simulink model "Transition"  (R2019a)
settings: Solver=VariableStepAuto  StartTime=0.0  StopTime=40  RelTol=1e-3
values from neighbouring files (symbols this model uses):
  agent = rlDDPGAgent(actor,critic,agentOptions)    [Agent.m]    (also in Bigger_Agent.m = agent.saved_agent; Multirotor_Agent.m = rlDDPGAgent(actor,critic,agentOpts); Transition_Agent.m = rlDDPGAgent(actor,critic,agentOpts))
  Ts = 0.4    [Agent.m]    (also in Bigger_Agent.m = 0.3; Multirotor_Agent.m = 0.3; Transition_Agent.m = 0.3)
libraries: simulink x14, simulink_extras x5, sharedutil x3, aerolibasang x2, shared6dof x1, aerolibadyn x1
(part 2 of 2)

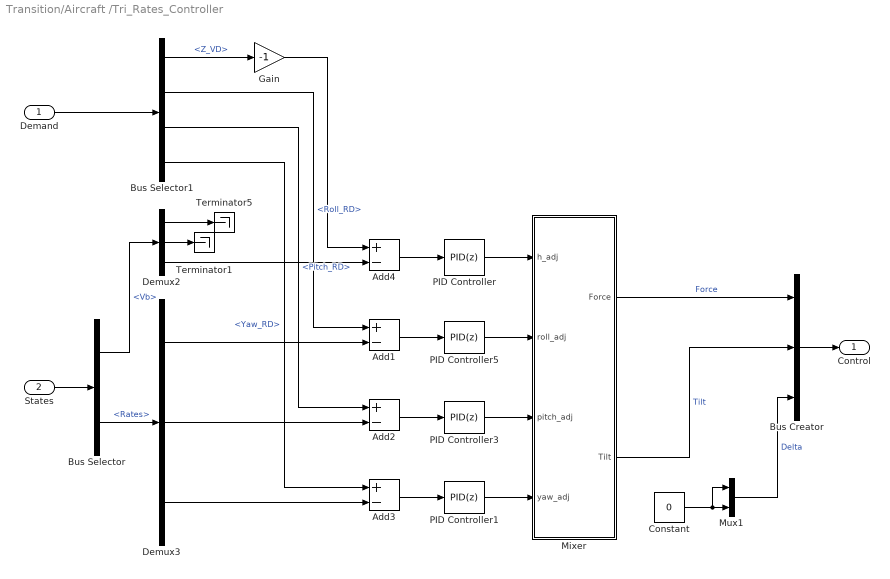
== system Transition/Aircraft /Tri_Rates_Controller ==
  Demand : Inport
  "States " : Inport  Port=2
  Add{1..4} (4 alike) : Sum  Inputs=+-
  Bus Creator : BusCreator  Inputs=3
  Bus Selector : BusSelector  OutputSignals=Vb,Rates
  Bus Selector1 : BusSelector  OutputSignals=Z_VD,Roll_RD,Pitch_RD,Yaw_RD
  Constant : Constant  Value=0
  Demux2 : Demux  Outputs=3
  Demux3 : Demux  Outputs=3
  Gain : Gain  Gain=-1
  Mixer : Subsystem
  Mux1 : Mux  Inputs=2
  PID Controller : simulink/Continuous/PID Controller  Controller=PID  Form=Parallel  TimeDomain=Discrete-time  SampleTime=0.001  IntegratorMethod=Forward Euler  FilterMethod=Forward Euler  ControllerParametersSource=internal  P=30  I=0.01  D=1  UseFilter=on  N=21.8158810168648  TunerSelectOption=Transfer Function Based (PID Tuner App)  InitialConditionSource=internal  InitialConditionForIntegrator=0  InitialConditionForFilter=0  DifferentiatorICPrevScaledInput=0  ExternalReset=none  TrackingMode=off  Kt=1  LimitOutput=off  UpperSaturationLimit=inf  LowerSaturationLimit=-inf  LinearizeAsGain=on  AntiWindupMode=none  Kb=1  POutMin=[]  POutMax=[]  IOutMin=[]  IOutMax=[]  DOutMin=[]  DOutMax=[]  NOutMin=[]  NOutMax=[]  SumOutMin=[]  SumOutMax=[]  SaturationOutMin=[]  SaturationOutMax=[]  PParamMin=[]  PParamMax=[]  IParamMin=[]  IParamMax=[]  DParamMin=[]  DParamMax=[]  NParamMin=[]  NParamMax=[]  KbParamMin=[]  KbParamMax=[]  KtParamMin=[]  KtParamMax=[]  KbOutMin=[]  KbOutMax=[]  KtOutMin=[]  KtOutMax=[]  IntegratorOutMin=[]  IntegratorOutMax=[]  FilterOutMin=[]  FilterOutMax=[]  SumI1OutMin=[]  SumI1OutMax=[]  SumI2OutMin=[]  SumI2OutMax=[]  SumI3OutMin=[]  SumI3OutMax=[]  SumI4OutMin=[]  SumI4OutMax=[]  SumDOutMin=[]  SumDOutMax=[]  DifferentiatorOutMin=[]  DifferentiatorOutMax=[]  FilterDiffOutCoefMin=[]  FilterDiffOutCoefMax=[]  ReciprocalOutMin=[]  ReciprocalOutMax=[]  SumDenOutMin=[]  SumDenOutMax=[]  SumNumOutMin=[]  SumNumOutMax=[]  DivideOutMin=[]  DivideOutMax=[]  IntegratorContinuousStateAttributes=''  IntegratorStateMustResolveToSignalObject=off  IntegratorRTWStateStorageClass=Auto  FilterContinuousStateAttributes=''  FilterStateMustResolveToSignalObject=off  FilterRTWStateStorageClass=Auto  ParallelPVariant=InternalParameters  IdealPVariant=Disabled  IVariant=InternalParameters  DVariant=InternalParameters  IntegratorVariant=Discrete  SatVariant=Disabled  AWVariant=Passthrough  PCopyVariant=Disabled  TRVariant=Disabled  FdbkBlocksVariant=Forward  IdealPFdbkVariant=Disabled  SatFdbkVariant=Disabled  DerivativeFilterVariant=ForwardEulerFilter  NVariant=InternalParameters  NCopyVariant=Disabled  FilterICVariant=InternalICsFilter  IntegratorICVariant=InternalICs  ExternalResetVariant=Disabled  TRSumVariant=Passthrough  SumFdbkVariant=Disabled  SumVariant=Sum_PID
  PID Controller1 : simulink/Continuous/PID Controller  Controller=PID  Form=Parallel  TimeDomain=Discrete-time  SampleTime=0.001  IntegratorMethod=Forward Euler  FilterMethod=Forward Euler  ControllerParametersSource=internal  P=30  I=0.01  D=2  UseFilter=on  N=200  TunerSelectOption=Transfer Function Based (PID Tuner App)  InitialConditionSource=internal  InitialConditionForIntegrator=0  InitialConditionForFilter=0  DifferentiatorICPrevScaledInput=0  ExternalReset=none  TrackingMode=off  Kt=1  LimitOutput=off  UpperSaturationLimit=inf  LowerSaturationLimit=-inf  LinearizeAsGain=on  AntiWindupMode=none  Kb=1  POutMin=[]  POutMax=[]  IOutMin=[]  IOutMax=[]  DOutMin=[]  DOutMax=[]  NOutMin=[]  NOutMax=[]  SumOutMin=[]  SumOutMax=[]  SaturationOutMin=[]  SaturationOutMax=[]  PParamMin=[]  PParamMax=[]  IParamMin=[]  IParamMax=[]  DParamMin=[]  DParamMax=[]  NParamMin=[]  NParamMax=[]  KbParamMin=[]  KbParamMax=[]  KtParamMin=[]  KtParamMax=[]  KbOutMin=[]  KbOutMax=[]  KtOutMin=[]  KtOutMax=[]  IntegratorOutMin=[]  IntegratorOutMax=[]  FilterOutMin=[]  FilterOutMax=[]  SumI1OutMin=[]  SumI1OutMax=[]  SumI2OutMin=[]  SumI2OutMax=[]  SumI3OutMin=[]  SumI3OutMax=[]  SumI4OutMin=[]  SumI4OutMax=[]  SumDOutMin=[]  SumDOutMax=[]  DifferentiatorOutMin=[]  DifferentiatorOutMax=[]  FilterDiffOutCoefMin=[]  FilterDiffOutCoefMax=[]  ReciprocalOutMin=[]  ReciprocalOutMax=[]  SumDenOutMin=[]  SumDenOutMax=[]  SumNumOutMin=[]  SumNumOutMax=[]  DivideOutMin=[]  DivideOutMax=[]  IntegratorContinuousStateAttributes=''  IntegratorStateMustResolveToSignalObject=off  IntegratorRTWStateStorageClass=Auto  FilterContinuousStateAttributes=''  FilterStateMustResolveToSignalObject=off  FilterRTWStateStorageClass=Auto  ParallelPVariant=InternalParameters  IdealPVariant=Disabled  IVariant=InternalParameters  DVariant=InternalParameters  IntegratorVariant=Discrete  SatVariant=Disabled  AWVariant=Passthrough  PCopyVariant=Disabled  TRVariant=Disabled  FdbkBlocksVariant=Forward  IdealPFdbkVariant=Disabled  SatFdbkVariant=Disabled  DerivativeFilterVariant=ForwardEulerFilter  NVariant=InternalParameters  NCopyVariant=Disabled  FilterICVariant=InternalICsFilter  IntegratorICVariant=InternalICs  ExternalResetVariant=Disabled  TRSumVariant=Passthrough  SumFdbkVariant=Disabled  SumVariant=Sum_PID
  PID Controller3 : simulink/Continuous/PID Controller  Controller=PID  Form=Parallel  TimeDomain=Discrete-time  SampleTime=0.001  IntegratorMethod=Forward Euler  FilterMethod=Forward Euler  ControllerParametersSource=internal  P=40  I=0.01  D=2  UseFilter=on  N=200  TunerSelectOption=Transfer Function Based (PID Tuner App)  InitialConditionSource=internal  InitialConditionForIntegrator=0  InitialConditionForFilter=0  DifferentiatorICPrevScaledInput=0  ExternalReset=none  TrackingMode=off  Kt=1  LimitOutput=off  UpperSaturationLimit=inf  LowerSaturationLimit=-inf  LinearizeAsGain=on  AntiWindupMode=none  Kb=1  POutMin=[]  POutMax=[]  IOutMin=[]  IOutMax=[]  DOutMin=[]  DOutMax=[]  NOutMin=[]  NOutMax=[]  SumOutMin=[]  SumOutMax=[]  SaturationOutMin=[]  SaturationOutMax=[]  PParamMin=[]  PParamMax=[]  IParamMin=[]  IParamMax=[]  DParamMin=[]  DParamMax=[]  NParamMin=[]  NParamMax=[]  KbParamMin=[]  KbParamMax=[]  KtParamMin=[]  KtParamMax=[]  KbOutMin=[]  KbOutMax=[]  KtOutMin=[]  KtOutMax=[]  IntegratorOutMin=[]  IntegratorOutMax=[]  FilterOutMin=[]  FilterOutMax=[]  SumI1OutMin=[]  SumI1OutMax=[]  SumI2OutMin=[]  SumI2OutMax=[]  SumI3OutMin=[]  SumI3OutMax=[]  SumI4OutMin=[]  SumI4OutMax=[]  SumDOutMin=[]  SumDOutMax=[]  DifferentiatorOutMin=[]  DifferentiatorOutMax=[]  FilterDiffOutCoefMin=[]  FilterDiffOutCoefMax=[]  ReciprocalOutMin=[]  ReciprocalOutMax=[]  SumDenOutMin=[]  SumDenOutMax=[]  SumNumOutMin=[]  SumNumOutMax=[]  DivideOutMin=[]  DivideOutMax=[]  IntegratorContinuousStateAttributes=''  IntegratorStateMustResolveToSignalObject=off  IntegratorRTWStateStorageClass=Auto  FilterContinuousStateAttributes=''  FilterStateMustResolveToSignalObject=off  FilterRTWStateStorageClass=Auto  ParallelPVariant=InternalParameters  IdealPVariant=Disabled  IVariant=InternalParameters  DVariant=InternalParameters  IntegratorVariant=Discrete  SatVariant=Disabled  AWVariant=Passthrough  PCopyVariant=Disabled  TRVariant=Disabled  FdbkBlocksVariant=Forward  IdealPFdbkVariant=Disabled  SatFdbkVariant=Disabled  DerivativeFilterVariant=ForwardEulerFilter  NVariant=InternalParameters  NCopyVariant=Disabled  FilterICVariant=InternalICsFilter  IntegratorICVariant=InternalICs  ExternalResetVariant=Disabled  TRSumVariant=Passthrough  SumFdbkVariant=Disabled  SumVariant=Sum_PID
  PID Controller5 : simulink/Continuous/PID Controller  Controller=PID  Form=Parallel  TimeDomain=Discrete-time  SampleTime=0.001  IntegratorMethod=Forward Euler  FilterMethod=Forward Euler  ControllerParametersSource=internal  P=20  I=0.01  D=2  UseFilter=on  N=200  TunerSelectOption=Transfer Function Based (PID Tuner App)  InitialConditionSource=internal  InitialConditionForIntegrator=0  InitialConditionForFilter=0  DifferentiatorICPrevScaledInput=0  ExternalReset=none  TrackingMode=off  Kt=1  LimitOutput=off  UpperSaturationLimit=inf  LowerSaturationLimit=-inf  LinearizeAsGain=on  AntiWindupMode=none  Kb=1  POutMin=[]  POutMax=[]  IOutMin=[]  IOutMax=[]  DOutMin=[]  DOutMax=[]  NOutMin=[]  NOutMax=[]  SumOutMin=[]  SumOutMax=[]  SaturationOutMin=[]  SaturationOutMax=[]  PParamMin=[]  PParamMax=[]  IParamMin=[]  IParamMax=[]  DParamMin=[]  DParamMax=[]  NParamMin=[]  NParamMax=[]  KbParamMin=[]  KbParamMax=[]  KtParamMin=[]  KtParamMax=[]  KbOutMin=[]  KbOutMax=[]  KtOutMin=[]  KtOutMax=[]  IntegratorOutMin=[]  IntegratorOutMax=[]  FilterOutMin=[]  FilterOutMax=[]  SumI1OutMin=[]  SumI1OutMax=[]  SumI2OutMin=[]  SumI2OutMax=[]  SumI3OutMin=[]  SumI3OutMax=[]  SumI4OutMin=[]  SumI4OutMax=[]  SumDOutMin=[]  SumDOutMax=[]  DifferentiatorOutMin=[]  DifferentiatorOutMax=[]  FilterDiffOutCoefMin=[]  FilterDiffOutCoefMax=[]  ReciprocalOutMin=[]  ReciprocalOutMax=[]  SumDenOutMin=[]  SumDenOutMax=[]  SumNumOutMin=[]  SumNumOutMax=[]  DivideOutMin=[]  DivideOutMax=[]  IntegratorContinuousStateAttributes=''  IntegratorStateMustResolveToSignalObject=off  IntegratorRTWStateStorageClass=Auto  FilterContinuousStateAttributes=''  FilterStateMustResolveToSignalObject=off  FilterRTWStateStorageClass=Auto  ParallelPVariant=InternalParameters  IdealPVariant=Disabled  IVariant=InternalParameters  DVariant=InternalParameters  IntegratorVariant=Discrete  SatVariant=Disabled  AWVariant=Passthrough  PCopyVariant=Disabled  TRVariant=Disabled  FdbkBlocksVariant=Forward  IdealPFdbkVariant=Disabled  SatFdbkVariant=Disabled  DerivativeFilterVariant=ForwardEulerFilter  NVariant=InternalParameters  NCopyVariant=Disabled  FilterICVariant=InternalICsFilter  IntegratorICVariant=InternalICs  ExternalResetVariant=Disabled  TRSumVariant=Passthrough  SumFdbkVariant=Disabled  SumVariant=Sum_PID
  Terminator1 : Terminator
  Terminator5 : Terminator
  Control : Outport
  wires:
  Add2/1 -> PID Controller3/1
  Add3/1 -> PID Controller1/1
  Add1/1 -> PID Controller5/1
  PID Controller5/1 -> Mixer/2(roll_adj)
  PID Controller1/1 -> Mixer/4(yaw_adj)
  PID Controller3/1 -> Mixer/3(pitch_adj)
  Mixer/2(Tilt) -> Bus Creator/2  "Tilt"
  Mux1/1 -> Bus Creator/3  "Delta"
  Bus Creator/1 -> Control/1
  Mixer/1(Force) -> Bus Creator/1  "Force"
  Constant/1 -> Mux1/2, Mux1/1
  Add4/1 -> PID Controller/1
  PID Controller/1 -> Mixer/1(h_adj)
  Bus Selector1/1 -> Gain/1  "<Z_VD>"
  Bus Selector1/3 -> Add2/1  "<Pitch_RD>"
  Bus Selector1/2 -> Add1/1  "<Roll_RD>"
  Demux2/3 -> Add4/2
  "States "/1 -> Bus Selector/1
  Bus Selector/2 -> Demux3/1  "<Rates>"
  Bus Selector/1 -> Demux2/1  "<Vb>"
  Demux3/1 -> Add1/2
  Demux3/2 -> Add2/2
  Demux3/3 -> Add3/2
  Demand/1 -> Bus Selector1/1
  Demux2/2 -> Terminator1/1
  Demux2/1 -> Terminator5/1
  Bus Selector1/4 -> Add3/1  "<Yaw_RD>"
  Gain/1 -> Add4/1

== system Transition/RL Agent/accumulate_reward ==
  reward : Inport
  Constant : Constant
  Unit Delay : UnitDelay  SampleTime=-1  HasFrameUpgradeWarning=on
  Zero-Order Hold : ZeroOrderHold  SampleTime=-1
  cumsum : Subsystem
  cumulative_reward : Outport
  wires:
  reward/1 -> Zero-Order Hold/1
  cumsum/1(cumulative_rwd) -> cumulative_reward/1
  Unit Delay/1 -> cumsum/Enable
  Constant/1 -> Unit Delay/1
  Zero-Order Hold/1 -> cumsum/1(rwd)

== system Transition/Subsystem1/-1//1 to 0//1_1 ==
  <i> : Inport
  Add : Sum
  Constant : Constant
  Gain : Gain  Gain=0.5
  o : Outport
  wires:
  Add/1 -> Gain/1
  <i>/1 -> Add/2
  Constant/1 -> Add/1
  Gain/1 -> o/1

== system Transition/Subsystem1/-1//1 to 0//1_2 ==
  <i> : Inport
  Add : Sum
  Constant : Constant
  Gain : Gain  Gain=0.5
  o : Outport
  wires:
  Add/1 -> Gain/1
  <i>/1 -> Add/2
  Constant/1 -> Add/1
  Gain/1 -> o/1

== system Transition/Subsystem1/-1//1 to 0//1_3 ==
  <i> : Inport
  Add : Sum
  Constant : Constant
  Gain : Gain  Gain=0.5
  o : Outport
  wires:
  Add/1 -> Gain/1
  <i>/1 -> Add/2
  Constant/1 -> Add/1
  Gain/1 -> o/1

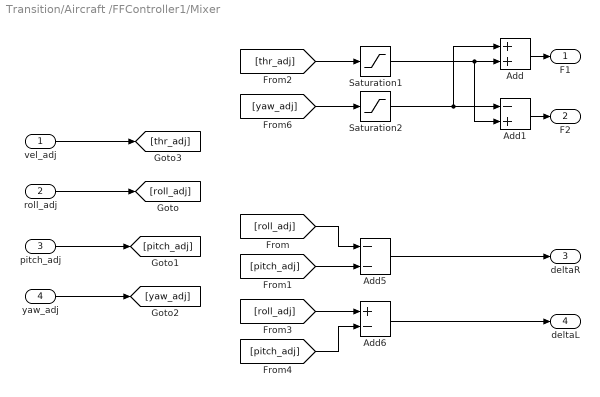
== system Transition/Aircraft /FFController1/Mixer ==
  vel_adj : Inport
  roll_adj : Inport  Port=2
  pitch_adj : Inport  Port=3
  yaw_adj : Inport  Port=4
  Add : Sum
  Add1 : Sum  Inputs=-+
  Add5 : Sum  Inputs=--
  Add6 : Sum  Inputs=+-
  Saturation1 : Saturate  UpperLimit=0.8  LowerLimit=0  ZeroCross=off
  Saturation2 : Saturate  UpperLimit=0.2  LowerLimit=0  ZeroCross=off
  F1 : Outport
  F2 : Outport  Port=2
  deltaR : Outport  Port=3
  deltaL : Outport  Port=4
  wires:
  Add5/1 -> deltaR/1
  roll_adj/1 -> [roll_adj]
  pitch_adj/1 -> [pitch_adj]
  [roll_adj] -> Add6/1
  [pitch_adj] -> Add5/2
  yaw_adj/1 -> [yaw_adj]
  [roll_adj] -> Add5/1
  [pitch_adj] -> Add6/2
  Add6/1 -> deltaL/1
  vel_adj/1 -> [thr_adj]
  [thr_adj] -> Saturation1/1
  Add/1 -> F1/1
  Add1/1 -> F2/1
  Saturation1/1 -> Add/2, Add1/2
  [yaw_adj] -> Saturation2/1
  Saturation2/1 -> Add1/1, Add/1

== system Transition/Aircraft /FF_Attitude Controller1/-1//1 to 0//1_1 ==
  <i> : Inport
  Add : Sum
  Constant : Constant
  Gain : Gain  Gain=0.5
  o : Outport
  wires:
  Add/1 -> Gain/1
  <i>/1 -> Add/2
  Constant/1 -> Add/1
  Gain/1 -> o/1

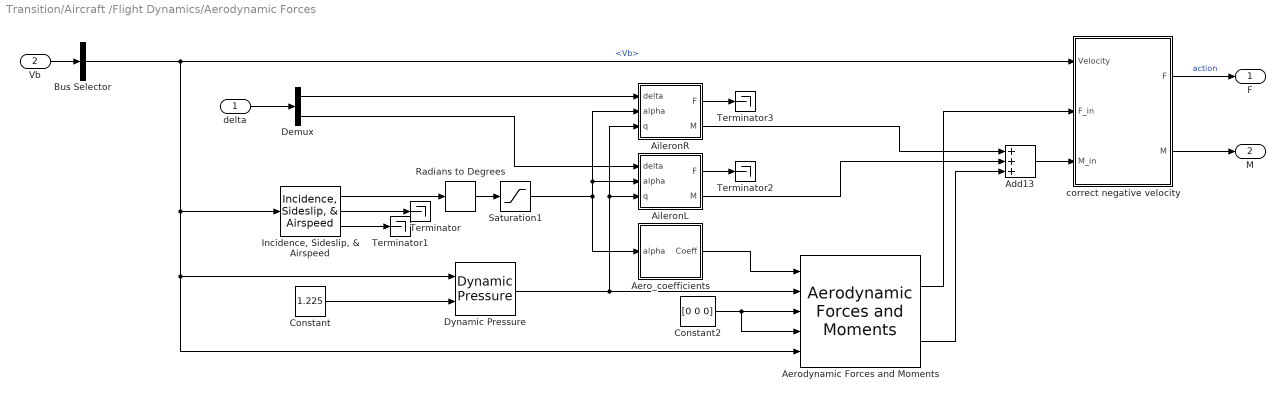
== system Transition/Aircraft /Flight Dynamics/Aerodynamic Forces ==
  delta : Inport
  Vb : Inport  Port=2
  Add13 : Sum  Inputs=+++
  Aero_coefficients : Subsystem
  "Aerodynamic Forces and Moments " : aerolibadyn/Aerodynamic Forces and Moments   inputAxes=Stability  outputForceAxes=Body  outputMomentAxes=Body  S=0.84  b=2.11  cbar=0.53
      settings: SourceProductName=Aerospace Blockset
  AileronL : Subsystem
  AileronR : Subsystem
  Bus Selector : BusSelector  OutputSignals=Vb
  Constant : Constant  Value=1.225
  Constant2 : Constant  Value=[0 0 0]
  Demux : Demux  Outputs=2
  Dynamic Pressure : aerolibasang/Dynamic Pressure
  "Incidence, Sideslip, & Airspeed" : aerolibasang/Incidence, Sideslip, & Airspeed
      settings: SourceProductName=Aerospace Blockset
  Radians to Degrees : simulink_extras/Transformations/Radians to Degrees
  Saturation1 : Saturate  UpperLimit=22  LowerLimit=-22  ZeroCross=off
  Terminator{,1..3} (4 alike) : Terminator
  correct negative velocity : MATLAB Function  TreatAsAtomicUnit=on
  F : Outport
  M : Outport  Port=2
  wires:
  Radians to Degrees/1 -> Saturation1/1
  Constant2/1 -> "Aerodynamic Forces and Moments "/4, "Aerodynamic Forces and Moments "/3
  Aero_coefficients/1(Coeff) -> "Aerodynamic Forces and Moments "/1
  "Incidence, Sideslip, & Airspeed"/1 -> Radians to Degrees/1
  Dynamic Pressure/1 -> "Aerodynamic Forces and Moments "/2, AileronR/3(q), AileronL/3(q)
  Constant/1 -> Dynamic Pressure/2
  Saturation1/1 -> AileronR/2(alpha), AileronL/2(alpha), Aero_coefficients/1(alpha)
  AileronL/2(M) -> Add13/2
  "Aerodynamic Forces and Moments "/2 -> Add13/3
  "Incidence, Sideslip, & Airspeed"/2 -> Terminator/1
  "Incidence, Sideslip, & Airspeed"/3 -> Terminator1/1
  correct negative velocity/1(F) -> F/1  "action"
  correct negative velocity/2(M) -> M/1
  Add13/1 -> correct negative velocity/3(M_in)
  "Aerodynamic Forces and Moments "/1 -> correct negative velocity/2(F_in)
  Vb/1 -> Bus Selector/1
  AileronR/2(M) -> Add13/1
  Bus Selector/1 -> "Incidence, Sideslip, & Airspeed"/1, "Aerodynamic Forces and Moments "/5, Dynamic Pressure/1, correct negative velocity/1(Velocity)  "<Vb>"
  delta/1 -> Demux/1
  Demux/1 -> AileronR/1(delta)
  Demux/2 -> AileronL/1(delta)
  AileronR/1(F) -> Terminator3/1
  AileronL/1(F) -> Terminator2/1

== system Transition/Aircraft /Flight Dynamics/Gravitational Forces ==
  states : Inport
  Bus Selector : BusSelector  OutputSignals=DCM
  Constant1 : Constant  Value=[0; 0; 9.81]
  Matrix Multiply : Product  Multiplication=Matrix(*)
  mass : Gain  Gain=mass
  Fg : Outport
  wires:
  Constant1/1 -> mass/1
  Matrix Multiply/1 -> Fg/1
  mass/1 -> Matrix Multiply/2
  Bus Selector/1 -> Matrix Multiply/1  "<DCM>"
  states/1 -> Bus Selector/1

== system Transition/Aircraft /Flight Dynamics/Propulsive Forces ==
  "F_M " : Inport
  Tilt : Inport  Port=2
  Add : Sum  Inputs=+++
  Add1 : Sum  Inputs=+++
  Demux : Demux  Outputs=3
  Demux1 : Demux  Outputs=2
  Gain : Gain  Gain=F
  Gain1 : Gain  Gain=F
  Gain2 : Gain  Gain=2*F
  force_moment_1 : Subsystem  mask{PoA=[-0.5, -0.5, 0]}
      mask prompts: PoA "point of action"
  force_moment_2 : Subsystem  mask{PoA=[-0.5, 0.5, 0]}
      mask prompts: PoA "point of action"
  force_moment_3 : Subsystem  mask{PoA=[0.5, 0, 0]}
      mask prompts: PoA "point of action"
  F : Outport
  M : Outport  Port=2
  wires:
  Add1/1 -> F/1
  Demux/1 -> Gain/1
  "F_M "/1 -> Demux/1
  Demux/2 -> Gain1/1
  Demux/3 -> Gain2/1
  Add/1 -> M/1
  Gain/1 -> force_moment_1/1(Force)
  force_moment_3/1(M3) -> Add/3
  force_moment_3/2(F3) -> Add1/3
  force_moment_1/1(M1) -> Add/1
  Demux1/1 -> force_moment_1/2(Tilt)
  Tilt/1 -> Demux1/1
  force_moment_1/2("F1 ") -> Add1/1
  force_moment_2/1(M2) -> Add/2
  Demux1/2 -> force_moment_2/2(Tilt)
  force_moment_2/2("F2 ") -> Add1/2
  Gain1/1 -> force_moment_2/1(Force)
  Gain2/1 -> force_moment_3/1(Force)

== system Transition/Aircraft /Subsystem1/Add ==
  in_ff : Inport
  in_tri : Inport  Port=2
  Tilt_offset : Inport  Port=3
  Add : Sum
  Add1 : Sum  Inputs=+++
  Add2 : Sum
  Bus Creator : BusCreator  Inputs=3
  Bus Selector1 : BusSelector  OutputSignals=Force,Tilt,Delta
  Bus Selector2 : BusSelector  OutputSignals=Force,Tilt,Delta
  Mux : Mux  Inputs=2
  Out1 : Outport
  wires:
  Add2/1 -> Bus Creator/3  "Delta"
  Bus Selector1/2 -> Add1/2  "<Tilt>"
  Bus Creator/1 -> Out1/1
  Bus Selector1/1 -> Add/2  "<Force>"
  Bus Selector1/3 -> Add2/2  "<Delta>"
  Add/1 -> Bus Creator/1  "Force"
  Add1/1 -> Bus Creator/2  "Tilt"
  in_tri/1 -> Bus Selector1/1
  in_ff/1 -> Bus Selector2/1
  Bus Selector2/3 -> Add2/1  "<Delta>"
  Bus Selector2/2 -> Add1/1  "<Tilt>"
  Bus Selector2/1 -> Add/1  "<Force>"
  Mux/1 -> Add1/3
  Tilt_offset/1 -> Mux/2, Mux/1

== system Transition/Aircraft /Subsystem1/Multiply_1 ==
  Weight : Inport
  Control_in : Inport  Port=2
  Bus Creator : BusCreator  Inputs=3
  Bus Selector1 : BusSelector  OutputSignals=Force,Tilt,Delta
  Product4 : Product
  Product5 : Product
  Product6 : Product
  Control_out : Outport
  wires:
  Weight/1 -> Product6/1, Product5/1, Product4/1
  Product5/1 -> Bus Creator/2  "Tilt"
  Bus Selector1/2 -> Product5/2  "<Tilt>"
  Bus Selector1/3 -> Product6/2  "<Delta>"
  Bus Creator/1 -> Control_out/1
  Product6/1 -> Bus Creator/3  "Delta"
  Control_in/1 -> Bus Selector1/1
  Product4/1 -> Bus Creator/1  "Force"
  Bus Selector1/1 -> Product4/2  "<Force>"

== system Transition/Aircraft /Subsystem1/Multiply_2 ==
  Weight : Inport
  Control_in : Inport  Port=2
  Bus Creator : BusCreator  Inputs=3
  Bus Selector1 : BusSelector  OutputSignals=Force,Tilt,Delta
  Product4 : Product
  Product5 : Product
  Product6 : Product
  Control_out : Outport
  wires:
  Weight/1 -> Product6/1, Product5/1, Product4/1
  Product5/1 -> Bus Creator/2  "Tilt"
  Bus Selector1/2 -> Product5/2  "<Tilt>"
  Bus Selector1/3 -> Product6/2  "<Delta>"
  Bus Creator/1 -> Control_out/1
  Product6/1 -> Bus Creator/3  "Delta"
  Control_in/1 -> Bus Selector1/1
  Product4/1 -> Bus Creator/1  "Force"
  Bus Selector1/1 -> Product4/2  "<Force>"

== system Transition/Aircraft /Tri_Attitude Controller/Subsystem ==
  Euler : Inport
  Demux1 : Demux  Outputs=3
  Roll : Outport
  Pitch : Outport  Port=2
  Yaw : Outport  Port=3
  wires:
  Euler/1 -> Demux1/1
  Demux1/3 -> Yaw/1
  Demux1/2 -> Pitch/1
  Demux1/1 -> Roll/1

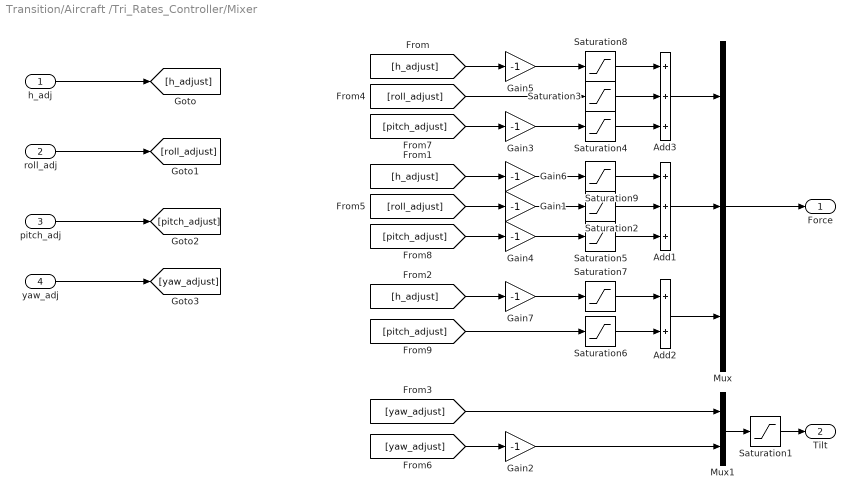
== system Transition/Aircraft /Tri_Rates_Controller/Mixer ==
  h_adj : Inport
  roll_adj : Inport  Port=2
  pitch_adj : Inport  Port=3
  yaw_adj : Inport  Port=4
  Add1 : Sum  Inputs=+++
  Add2 : Sum
  Add3 : Sum  Inputs=+++
  Gain{1..7} (7 alike) : Gain  Gain=-1
  Mux : Mux  Inputs=3
  Mux1 : Mux  Inputs=2
  Saturation1 : Saturate  UpperLimit=2  LowerLimit=-2  ZeroCross=off
  Saturation{2..6} (5 alike) : Saturate  UpperLimit=0.3  LowerLimit=0  ZeroCross=off
  Saturation7 : Saturate  UpperLimit=0.7  LowerLimit=0  ZeroCross=off
  Saturation8 : Saturate  UpperLimit=0.7  LowerLimit=0  ZeroCross=off
  Saturation9 : Saturate  UpperLimit=0.7  LowerLimit=0  ZeroCross=off
  Force : Outport
  Tilt : Outport  Port=2
  wires:
  yaw_adj/1 -> [yaw_adjust]
  roll_adj/1 -> [roll_adjust]
  pitch_adj/1 -> [pitch_adjust]
  [roll_adjust] -> Gain1/1
  [pitch_adjust] -> Gain4/1
  Add3/1 -> Mux/1
  Add1/1 -> Mux/2
  [pitch_adjust] -> Gain3/1
  Mux/1 -> Force/1
  h_adj/1 -> [h_adjust]
  [yaw_adjust] -> Gain2/1
  Mux1/1 -> Saturation1/1
  Saturation1/1 -> Tilt/1
  [yaw_adjust] -> Mux1/1
  [h_adjust] -> Gain5/1
  [roll_adjust] -> Saturation3/1
  Gain3/1 -> Saturation4/1
  [h_adjust] -> Gain6/1
  [h_adjust] -> Gain7/1
  Gain1/1 -> Saturation2/1
  Gain4/1 -> Saturation5/1
  [pitch_adjust] -> Saturation6/1
  Gain2/1 -> Mux1/2
  Saturation2/1 -> Add1/2
  Saturation3/1 -> Add3/2
  Saturation4/1 -> Add3/3
  Saturation5/1 -> Add1/3
  Saturation6/1 -> Add2/2
  Add2/1 -> Mux/3
  Gain5/1 -> Saturation8/1
  Gain6/1 -> Saturation9/1
  Gain7/1 -> Saturation7/1
  Saturation7/1 -> Add2/1
  Saturation9/1 -> Add1/1
  Saturation8/1 -> Add3/1

== system Transition/RL Agent/accumulate_reward/cumsum ==
  rwd : Inport
  Enable : EnablePort
  Sum : Sum  Inputs=|++
  Unit Delay : UnitDelay  SampleTime=-1  HasFrameUpgradeWarning=on
  cumulative_rwd : Outport
  wires:
  rwd/1 -> Sum/1
  Sum/1 -> Unit Delay/1, cumulative_rwd/1
  Unit Delay/1 -> Sum/2

== system Transition/Aircraft /Flight Dynamics/Aerodynamic Forces/Aero_coefficients ==
  alpha : Inport
  Cd : Lookup_n-D  NumberOfTableDimensions=1  BreakpointsForDimension1=|  Table=|  InternalRulePriority=Speed  RndMeth=Simplest  InputSameDT=on
      BreakpointsForDimension1=|
      | [-22
      | -20
      | -18
      | -16
      | -14
      | -12
      | -10
      | -8
      | -6
      | -4
      | -2
      | 0
      | 2
      | 4
      | 6
      | 8
      | 10
      | 12
      | 14
      | 16
      | 18
      | 20
      | 22]
      Table=|
      | [0.392965675000000
      | 0.341758938000000
      | 0.291869622000000
      | 0.243198735000000
      | 0.201122935000000
      | 0.162088921000000
      | 0.119255102000000
      | 0.0879271140000000
      | 0.0661394560000000
      | 0.0508236150000000
      | 0.0422907190000000
      | 0.0388286200000000
      | 0.0390186100000000
      | 0.0428645290000000
      | 0.0503231290000000
      | 0.0617672500000000
      | 0.0796637510000000
      | 0.103830904000000
      | 0.130929057000000
      | 0.163534014000000
      | 0.205122935000000
      | 0.273406040000000
      | 0.340174273000000]
  Cl : Constant  Value=0
  "Cl " : Lookup_n-D  NumberOfTableDimensions=1  BreakpointsForDimension1=|  Table=|  InternalRulePriority=Speed  RndMeth=Simplest  InputSameDT=on
      BreakpointsForDimension1=|
      | [-22
      | -20
      | -18
      | -16
      | -14
      | -12
      | -10
      | -8
      | -6
      | -4
      | -2
      | 0
      | 2
      | 4
      | 6
      | 8
      | 10
      | 12
      | 14
      | 16
      | 18
      | 20
      | 22]
      Table=|
      | [-1.05304747000000
      | -0.939866144000000
      | -0.835877820000000
      | -0.772327502000000
      | -0.744091351000000
      | -0.678260447000000
      | -0.627152575000000
      | -0.541724976000000
      | -0.430579689000000
      | -0.309313897000000
      | -0.176928086000000
      | -0.0384528670000000
      | 0.102475219000000
      | 0.243855685000000
      | 0.381506317000000
      | 0.522103984000000
      | 0.649275996000000
      | 0.776705539000000
      | 0.874480078000000
      | 0.954319728000000
      | 1.00194617500000
      | 0.976721554000000
      | 0.991607470000000]
  Cm : Lookup_n-D  NumberOfTableDimensions=1  BreakpointsForDimension1=|  Table=|  InternalRulePriority=Speed  RndMeth=Simplest  InputSameDT=on
      BreakpointsForDimension1=|
      | [-22
      | -20
      | -18
      | -16
      | -14
      | -12
      | -10
      | -8
      | -6
      | -4
      | -2
      | 0
      | 2
      | 4
      | 6
      | 8
      | 10
      | 12
      | 14
      | 16
      | 18
      | 20
      | 22]
      Table=|
      | [-0.0374352130000000
      | -0.0346318370000000
      | -0.0299414270000000
      | -0.0257262990000000
      | -0.0215954230000000
      | -0.0114725440000000
      | 0.0141471030000000
      | 0.0288031780000000
      | 0.0376529660000000
      | 0.0436490160000000
      | 0.0450585630000000
      | 0.0429304540000000
      | 0.0377977440000000
      | 0.0321134120000000
      | 0.0258494080000000
      | 0.0177846340000000
      | 0.0110621100000000
      | 0.00550642000000000
      | 0.00100000000000000
      | -0.00339548100000000
      | 0.0115161200000000
      | 0.0292985040000000
      | 0.0374352130000000]
  Mux : Mux  Inputs=6
  Coeff : Outport
  wires:
  alpha/1 -> Cd/1, Cm/1, "Cl "/1
  Mux/1 -> Coeff/1
  Cd/1 -> Mux/1
  Cm/1 -> Mux/5
  "Cl "/1 -> Mux/3
  Cl/1 -> Mux/4, Mux/6, Mux/2

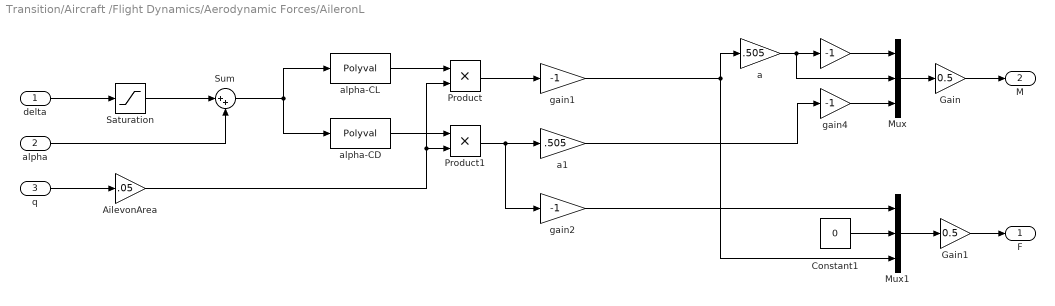
== system Transition/Aircraft /Flight Dynamics/Aerodynamic Forces/AileronL ==
  delta : Inport
  alpha : Inport  Port=2
  q : Inport  Port=3
  " " : Gain  Gain=-1
  AilevonArea : Gain  Gain=.05
  Constant1 : Constant  Value=0
  Gain : Gain  Gain=0.5
  Gain1 : Gain  Gain=0.5
  Mux : Mux  Inputs=3
  Mux1 : Mux  Inputs=3
  Product : Product
  Product1 : Product
  Saturation : Saturate  UpperLimit=20  LowerLimit=-20  ZeroCross=off
  Sum : Sum  Inputs=|++
  a : Gain  Gain=.505
  a1 : Gain  Gain=.505
  alpha-CD : Polyval  Coefs=[2e-5 2e-8 -5e-5 -4e-7 .0119]
  alpha-CL : Polyval  Coefs=[0.0987 0]
  gain1 : Gain  Gain=-1
  gain2 : Gain  Gain=-1
  gain4 : Gain  Gain=-1
  F : Outport
  M : Outport  Port=2
  wires:
  gain1/1 -> a/1, Mux1/3
  Product1/1 -> gain2/1, a1/1
  delta/1 -> Saturation/1
  AilevonArea/1 -> Product1/2, Product/2
  Sum/1 -> alpha-CL/1, alpha-CD/1
  a/1 -> Mux/2, " "/1
  gain2/1 -> Mux1/1
  Mux1/1 -> Gain1/1
  a1/1 -> gain4/1
  Product/1 -> gain1/1
  Constant1/1 -> Mux1/2
  Mux/1 -> Gain/1
  alpha-CL/1 -> Product/1
  alpha-CD/1 -> Product1/1
  alpha/1 -> Sum/2
  " "/1 -> Mux/1
  gain4/1 -> Mux/3
  Saturation/1 -> Sum/1
  q/1 -> AilevonArea/1
  Gain/1 -> M/1
  Gain1/1 -> F/1

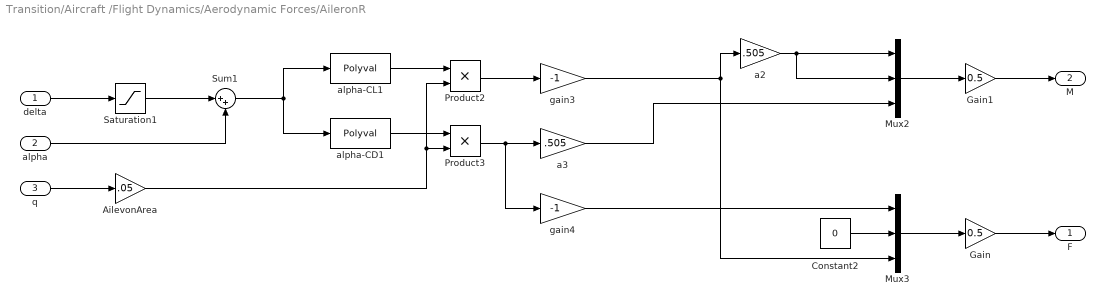
== system Transition/Aircraft /Flight Dynamics/Aerodynamic Forces/AileronR ==
  delta : Inport
  alpha : Inport  Port=2
  q : Inport  Port=3
  AilevonArea : Gain  Gain=.05
  Constant2 : Constant  Value=0
  Gain : Gain  Gain=0.5
  Gain1 : Gain  Gain=0.5
  Mux2 : Mux  Inputs=3
  Mux3 : Mux  Inputs=3
  Product2 : Product
  Product3 : Product
  Saturation1 : Saturate  UpperLimit=20  LowerLimit=-20  ZeroCross=off
  Sum1 : Sum  Inputs=|++
  a2 : Gain  Gain=.505
  a3 : Gain  Gain=.505
  alpha-CD1 : Polyval  Coefs=[2e-5 2e-8 -5e-5 -4e-7 .0119]
  alpha-CL1 : Polyval  Coefs=[0.0987 0]
  gain3 : Gain  Gain=-1
  gain4 : Gain  Gain=-1
  F : Outport
  M : Outport  Port=2
  wires:
  Saturation1/1 -> Sum1/1
  Product2/1 -> gain3/1
  a2/1 -> Mux2/1, Mux2/2
  alpha-CD1/1 -> Product3/1
  alpha/1 -> Sum1/2
  Sum1/1 -> alpha-CL1/1, alpha-CD1/1
  Product3/1 -> gain4/1, a3/1
  Mux3/1 -> Gain/1
  gain4/1 -> Mux3/1
  AilevonArea/1 -> Product3/2, Product2/2
  alpha-CL1/1 -> Product2/1
  gain3/1 -> a2/1, Mux3/3
  Constant2/1 -> Mux3/2
  q/1 -> AilevonArea/1
  delta/1 -> Saturation1/1
  Mux2/1 -> Gain1/1
  a3/1 -> Mux2/3
  Gain1/1 -> M/1
  Gain/1 -> F/1

== system Transition/Aircraft /Flight Dynamics/Propulsive Forces/force_moment_1 ==
  Force : Inport
  Tilt : Inport  Port=2
  3x3 Cross Product1 : sharedutil/3x3 Cross Product  aMode=aMode
      settings: SourceProductBaseCode=AE
  Constant1 : Constant  Value=0
  Cos : Trigonometry  Operator=cos
  Degrees to Radians : simulink_extras/Transformations/Degrees to Radians
  Gain3 : Gain  Gain=-1
  Mux2 : Mux  Inputs=3
  Product : Product
  Product1 : Product
  Trigonometric Function : Trigonometry
  point_of_action : Constant  Value=PoA  VectorParams1D=off
  M1 : Outport
  "F1 " : Outport  Port=2
  wires:
  Constant1/1 -> Mux2/2
  Product1/1 -> Mux2/3
  Tilt/1 -> Degrees to Radians/1
  Product/1 -> Mux2/1
  Trigonometric Function/1 -> Product/1
  Cos/1 -> Gain3/1
  Gain3/1 -> Product1/1
  Force/1 -> Product1/2, Product/2
  Mux2/1 -> "F1 "/1, 3x3 Cross Product1/2
  point_of_action/1 -> 3x3 Cross Product1/1
  3x3 Cross Product1/1 -> M1/1
  Degrees to Radians/1 -> Cos/1, Trigonometric Function/1

== system Transition/Aircraft /Flight Dynamics/Propulsive Forces/force_moment_2 ==
  Force : Inport
  Tilt : Inport  Port=2
  3x3 Cross Product1 : sharedutil/3x3 Cross Product  aMode=aMode
      settings: SourceProductBaseCode=AE
  Constant1 : Constant  Value=0
  Cos : Trigonometry  Operator=cos
  Degrees to Radians : simulink_extras/Transformations/Degrees to Radians
  Gain3 : Gain  Gain=-1
  Mux2 : Mux  Inputs=3
  Product : Product
  Product1 : Product
  Trigonometric Function : Trigonometry
  point_of_action : Constant  Value=PoA  VectorParams1D=off
  M2 : Outport
  "F2 " : Outport  Port=2
  wires:
  Constant1/1 -> Mux2/2
  Product1/1 -> Mux2/3
  Tilt/1 -> Degrees to Radians/1
  Product/1 -> Mux2/1
  Trigonometric Function/1 -> Product/1
  Cos/1 -> Gain3/1
  Gain3/1 -> Product1/1
  Force/1 -> Product1/2, Product/2
  Mux2/1 -> "F2 "/1, 3x3 Cross Product1/2
  point_of_action/1 -> 3x3 Cross Product1/1
  3x3 Cross Product1/1 -> M2/1
  Degrees to Radians/1 -> Cos/1, Trigonometric Function/1

== system Transition/Aircraft /Flight Dynamics/Propulsive Forces/force_moment_3 ==
  Force : Inport
  3x3 Cross Product : sharedutil/3x3 Cross Product  aMode=aMode
      settings: SourceProductBaseCode=AE
  Constant3 : Constant  Value=0
  Gain : Gain  Gain=-1
  Matrix Concatenate : Concatenate  NumInputs=3  ConcatenateDimension=2
  point_of_action2 : Constant  Value=PoA  VectorParams1D=off
  M3 : Outport
  F3 : Outport  Port=2
  wires:
  3x3 Cross Product/1 -> M3/1
  Constant3/1 -> Matrix Concatenate/2, Matrix Concatenate/1
  point_of_action2/1 -> 3x3 Cross Product/1
  Matrix Concatenate/1 -> F3/1, 3x3 Cross Product/2
  Gain/1 -> Matrix Concatenate/3
  Force/1 -> Gain/1

== matlab function Transition/Aircraft /Flight Dynamics/Aerodynamic Forces/correct negative velocity ==
  data: F output; Velocity input; F_in input; M_in input; M output
function [F,M] = Update(Velocity,F_in,M_in)  
    if Velocity(1) < 0
        F = [0;0;0];
        M = [0;0;0];
    else
        F = F_in;
        M = M_in;
    end
end

== matlab function Transition/MATLAB Function2 ==
  data: Tri_weight input; Tilt_offset input; Velocity input; weight output; offset output
function [weight,offset] = fcn(Tri_weight, Tilt_offset, Velocity)
    if Velocity(1) <8
        weight = 1;
        if Tilt_offset > 30
            offset = 30;
        else
            offset = Tilt_offset;
        end
    else
        weight = Tri_weight;
        offset = Tilt_offset;
    end
end
